simulink model "Pod_trav_plant_linear"  (R2022b)
settings: Solver=VariableStepAuto  StartTime=0.0  StopTime=10.0  RelTol=1e-3
undefined symbols (not defined in the file): fix_constt, JLrtg, JLrtt, JMrtg, JMrtt, Kktt, Kvtt
libraries: slctrlblks x1
settings Model: Creator=ohadformanair  LastModifiedBy=ohadformanair

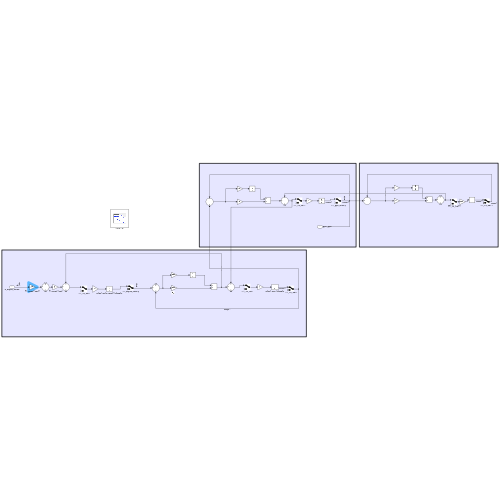
[thumbnail: Simulink's stored preview of the top-level diagram]
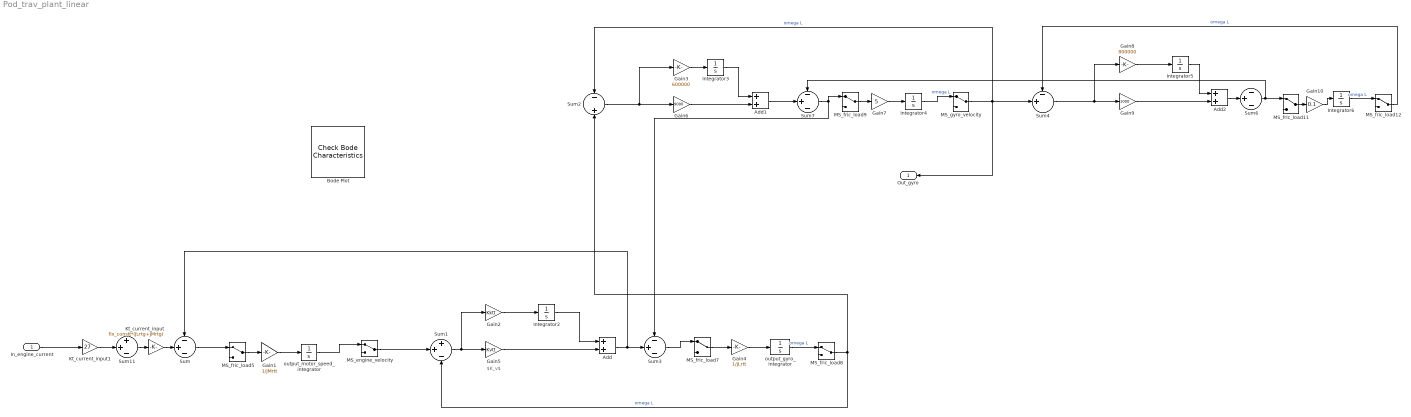
== system Pod_trav_plant_linear ==
  note: $K_v$
  In_engine_current : Inport
  Add : Sum
  Add1 : Sum
  Add2 : Sum
  Bode Plot : slctrlblks/Model Verification/Check Bode  Characteristics  InstantiateOnLoad=on  SaveOperatingPoints=off  LinearizationIOs={'/In_engine_current', 1, 'in', 'off', '';'/MS_engine_velocity', 1, 'out', 'off', '';'/MS_gyro_velocity', 1, 'out', 'off', ''}  LinearizeAt=SnapshotTimes  SnapshotTimes=[0]  TriggerType=rising  SampleTime=auto  RateConversionMethod=zoh  PreWarpFreq=10  UseExactDelayModel=off  UseFullBlockNameLabels=off  UseBusSignalLabels=off  enabled=on  stopWhenAssertionFail=off  export=off  ViewDlgPos=[]  OpenViewOnLoad=off  LaunchViewOnOpen=off  FrequencyUnits=Hz  MagnitudeUnits=dB  PhaseUnits=deg  TimeUnits=seconds  EnableUpperBound=off  UpperBoundFrequencies=[]  UpperBoundMagnitudes=[]  EnableLowerBound=off  LowerBoundFrequencies=[]  LowerBoundMagnitudes=[]
      settings: LibrarySourceBlock=slctrlblks/Linear Analysis Plots/Bode Plot
  Gain1 : Gain  Gain=1/JMrtt
  Gain10 : Gain  Gain=0.1
  Gain2 : Gain  Gain=Kktt
  Gain3 : Gain  Gain=600000
  Gain4 : Gain  Gain=1/JLrtt
  Gain5 : Gain  Gain=Kvtt
  Gain6 : Gain  Gain=9000
  Gain7 : Gain  Gain=5
  Gain8 : Gain  Gain=800000
  Gain9 : Gain  Gain=1000
  Integrator{2..6} (5 alike) : Integrator
  Kt_current_input : Gain  Gain=fix_constt*(JLrtg+JMrtg)
  Kt_current_input1 : Gain  Gain=27
  MS_engine_velocity : ManualSwitch
  MS_fric_load{5,7..9,11..12} (6 alike) : ManualSwitch
  MS_gyro_velocity : ManualSwitch
  Sum{,3,6..7} (4 alike) : Sum  Inputs=-+-
  Sum1 : Sum  Inputs=++-
  Sum11 : Sum  Inputs=++-
  Sum2 : Sum  Inputs=-+
  Sum4 : Sum  Inputs=-+|
  output_gyro_integrator : Integrator
  output_motor_speed_integrator : Integrator
  Out_gyro : Outport
  wires:
  Gain7/1 -> Integrator4/1
  Gain1/1 -> output_motor_speed_integrator/1
  Integrator5/1 -> Add2/1
  Integrator6/1 -> MS_fric_load12/1  "omega L"
  MS_gyro_velocity/1 -> Out_gyro/1, Sum2/1, Sum4/2  "omega L"
  MS_fric_load9/1 -> Gain7/1
  output_motor_speed_integrator/1 -> MS_engine_velocity/1
  Sum11/1 -> Kt_current_input/1
  Sum7/1 -> MS_fric_load9/1, Sum3/1
  Gain8/1 -> Integrator5/1
  Sum3/1 -> MS_fric_load7/1
  Gain3/1 -> Integrator3/1
  Gain4/1 -> output_gyro_integrator/1
  Kt_current_input/1 -> Sum/2
  MS_fric_load8/1 -> Sum1/3, Sum2/2  "omega L"
  Gain6/1 -> Add1/2
  Integrator3/1 -> Add1/1
  Gain5/1 -> Add/2
  Integrator2/1 -> Add/1
  Integrator4/1 -> MS_gyro_velocity/1  "omega L"
  Gain2/1 -> Integrator2/1
  Sum6/1 -> Sum7/1, MS_fric_load11/1
  Sum/1 -> MS_fric_load5/1
  MS_engine_velocity/1 -> Sum1/2
  Gain9/1 -> Add2/2
  Sum2/1 -> Gain6/1, Gain3/1
  Sum4/1 -> Gain9/1, Gain8/1
  MS_fric_load5/1 -> Gain1/1
  Gain10/1 -> Integrator6/1
  Sum1/1 -> Gain2/1, Gain5/1
  Add1/1 -> Sum7/2
  Add/1 -> Sum3/2, Sum/1
  output_gyro_integrator/1 -> MS_fric_load8/1  "omega L"
  Add2/1 -> Sum6/2
  MS_fric_load12/1 -> Sum4/1  "omega L"
  MS_fric_load11/1 -> Gain10/1
  MS_fric_load7/1 -> Gain4/1
  In_engine_current/1 -> Kt_current_input1/1
  Kt_current_input1/1 -> Sum11/2
